simulink model "FIR_Model"  (R2020a)
settings: Solver=VariableStepAuto  StartTime=0.0  StopTime=10.0  RelTol=1e-3
settings Model: Creator=DELL  LastModifiedBy=DELL
settings DataIOCC: SaveOutput=off  SaveTime=off

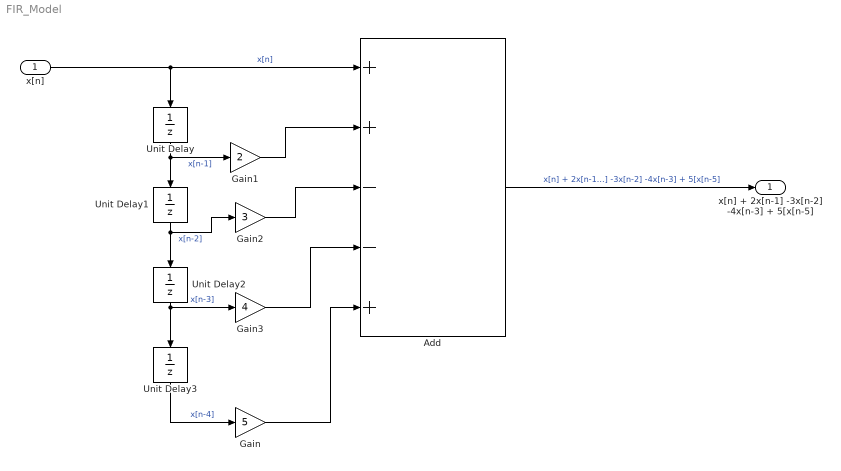
== system FIR_Model ==
  x[n] : Inport  OutDataTypeStr=double  PortDimensions=1  SampleTime=[0,1]
  Add : Sum  Inputs=++--+
  Gain : Gain  Gain=5
  Gain1 : Gain  Gain=2
  Gain2 : Gain  Gain=3
  Gain3 : Gain  Gain=4
  Unit Delay{,1..3} (4 alike) : UnitDelay  SampleTime=-1  HasFrameUpgradeWarning=on
  x[n] + 2x[n-1] -3x[n-2] -4x[n-3] + 5[x[n-5] : Outport  OutDataTypeStr=double  PortDimensions=1  SampleTime=[0,1]
  wires:
  Gain3/1 -> Add/4
  Unit Delay/1 -> Unit Delay1/1, Gain1/1  "x[n-1]"
  Gain1/1 -> Add/2
  Unit Delay1/1 -> Unit Delay2/1, Gain2/1  "x[n-2]"
  Gain2/1 -> Add/3
  Add/1 -> x[n] + 2x[n-1] -3x[n-2] -4x[n-3] + 5[x[n-5]/1  "x[n] + 2x[n-1] -3x[n-2] -4x[n-3] + 5[x[n-5]"
  x[n]/1 -> Add/1, Unit Delay/1  "x[n]"
  Unit Delay2/1 -> Gain3/1, Unit Delay3/1  "x[n-3]"
  Unit Delay3/1 -> Gain/1  "x[n-4]"
  Gain/1 -> Add/5
